simulink model "part16"  (R2020a)
settings: Solver=VariableStepAuto  StartTime=0.0  StopTime=40.0  RelTol=1e-3
settings Model: Creator=emami  LastModifiedBy=emami

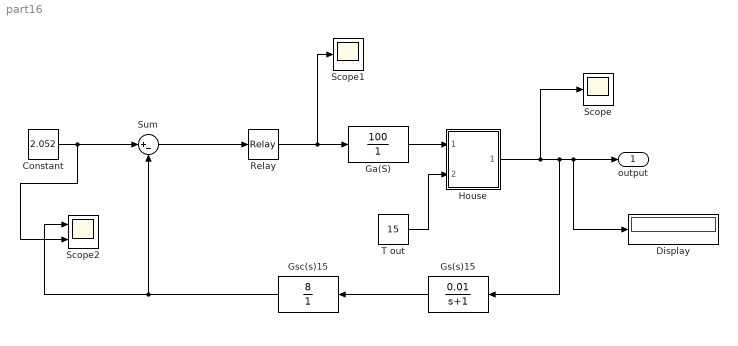
== system part16 ==
  " Gs(s)15" : TransferFcn  Numerator=[0.01]  Denominator=[1 1]
  " Gsc(s)15" : TransferFcn  Numerator=[8]  Denominator=[1]
  Constant : Constant  Value=2.052
  Display : Display
  Ga(S) : TransferFcn  Numerator=[100]  Denominator=[1]
  House : Subsystem
      mask Display: image(fullfile(matlabroot,'toolbox','simulink','simdemos','simgeneral','images','HouseHeatHousePix.svg'))
  Relay : Relay  OnSwitchValue=0.001  OffSwitchValue=-0.001  OnOutputValue=10
  Scope : Scope
  Scope1 : Scope
  Scope2 : Scope  NumInputPorts=2
  Sum : Sum  Inputs=|+-
  T out : Constant  Value=15
  output : Outport
  wires:
  T out/1 -> House/2(Outdoor Temp Tout)
  " Gsc(s)15"/1 -> Scope2/1, Sum/2
  " Gs(s)15"/1 -> " Gsc(s)15"/1
  Ga(S)/1 -> House/1(Heater QDot In)
  House/1(Room Temp Troom) -> Scope/1, " Gs(s)15"/1, Display/1, output/1
  Sum/1 -> Relay/1
  Relay/1 -> Scope1/1, Ga(S)/1
  Constant/1 -> Scope2/2, Sum/1

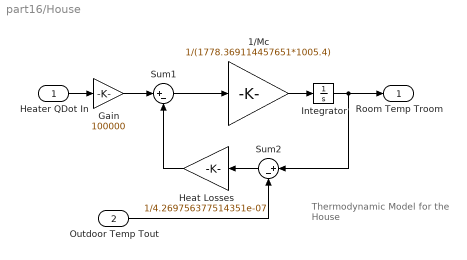
== system part16/House ==
  note: Thermodynamic Model
      | for the House
  Heater QDot In : Inport
  Outdoor Temp Tout : Inport  Port=2
  1/Mc : Gain  Gain=1/(1778.369114457651*1005.4)  SaturateOnIntegerOverflow=on  OutDataTypeStr=Inherit: Same as input  ParamDataTypeStr=Inherit: Same as input
  Gain : Gain  Gain=100000
  Heat Losses : Gain  Gain=1/4.269756377514351e-07  SaturateOnIntegerOverflow=on  OutDataTypeStr=Inherit: Same as input  ParamDataTypeStr=Inherit: Same as input
  Integrator : Integrator  InitialCondition=20
  Sum1 : Sum  Inputs=|+-  InputSameDT=on  SaturateOnIntegerOverflow=on  OutDataTypeStr=Inherit: Same as first input
  Sum2 : Sum  Inputs=|+-  InputSameDT=on  SaturateOnIntegerOverflow=on  OutDataTypeStr=Inherit: Same as first input
  Room Temp Troom : Outport  InitialOutput=0
  wires:
  Outdoor Temp Tout/1 -> Sum2/2
  Heater QDot In/1 -> Gain/1
  Sum1/1 -> 1/Mc/1
  Sum2/1 -> Heat Losses/1
  Heat Losses/1 -> Sum1/2
  1/Mc/1 -> Integrator/1
  Integrator/1 -> Sum2/1, Room Temp Troom/1
  Gain/1 -> Sum1/1
